simulink model "WK4_FOCIM"  (R2019b)
settings: Solver=VariableStepAuto  StartTime=0.0  StopTime=120.0  MaxStep=1/10000  RelTol=1e-3
values from neighbouring files (symbols this model uses):
  Bm = 15.1e-4    (= 0.00151)    [LAB_FOCIM_sim.m]    (also in LABprep.m; PMAC_machine.m = 7.59908877318e-07; WK1L1_DCmachine.m = Bm_init + Tmax*(i/10)*0.01; WK2_InductionMachine.m = 0.0337986596081)
  CurrentController = tf([133],[1 0])    [LAB_FOCIM_sim.m]    (also in WK4_FOCIM_mScript.m = tf([50],[1 0]))
  Is = 6.3    [LAB_FOCIM_sim.m]    (also in WK4_FOCIM_mScript.m)
  J = 27.6e-3    (= 0.0276)    [LAB_FOCIM_sim.m]    (also in LABprep.m; PMAC_machine.m = 2.55e-08; WK1L1_DCmachine.m = 0.134; WK2_InductionMachine.m = 0.0068)
  La = ((1/Lm)+(1/Lls)+(1/Llrd))^-1    (= 0.0046720399295)    [LAB_FOCIM_sim.m]    (also in LABprep.m = 0.0043; WK2_InductionMachine.m = 0.00475247524752; WK2_InductionMachine_LAB.m = 7.87664870863e-06; WK4_FOCIM_mScript.m = 0.00474852546917)
  Llrd = 11.82e-3    (= 0.01182)    [LAB_FOCIM_sim.m]    (also in WK2_InductionMachine.m = 0.012; WK2_InductionMachine_LAB.m; WK4_FOCIM_mScript.m = 0.012)
  Lls = 7.822*10^-3    (= 0.007822)    [LAB_FOCIM_sim.m]    (also in LABprep.m = 0.007882; PMAC_machine.m = 7.2e-06; WK2_InductionMachine.m = 0.008; WK2_InductionMachine_LAB.m = 7.882e-06)
  Lm = 0.628    [LAB_FOCIM_sim.m]    (also in LABprep.m; PMAC_machine.m = 6.48e-05; WK2_InductionMachine.m = 0.48; WK2_InductionMachine_LAB.m)
  LM_est = 0.9*Lrd_est    (= 0.4428)    [WK4_FOCIM_mScript.m]
  Lrd = Lm + Llrd    (= 0.63982)    [LAB_FOCIM_sim.m]    (also in LABprep.m; WK4_FOCIM_mScript.m = 0.492)
  Lrd_est = Lrd    (= 0.492)    [WK4_FOCIM_mScript.m]
  P = 2    [LAB_FOCIM_sim.m]    (also in PMAC_machine.m; WK2_InductionMachine.m; WK2_InductionMachine_LAB.m; WK4_FOCIM_mScript.m)
  refSpeed = 20    [WK4_FOCIM_mScript.m]
  rrd = 1.868    [LAB_FOCIM_sim.m]    (also in WK2_InductionMachine.m = 1.7; WK2_InductionMachine_LAB.m; WK4_FOCIM_mScript.m = 1.7)
  rs = 1.72    [LAB_FOCIM_sim.m]    (also in WK2_InductionMachine.m = 2; WK2_InductionMachine_LAB.m; WK4_FOCIM_mScript.m = 2)
  SpeedController = tf([0.166],[1 0])    [LAB_FOCIM_sim.m]    (also in WK4_FOCIM_mScript.m)
  w = 0    [LAB_FOCIM_sim.m]    (also in WK2_InductionMachine.m; WK2_InductionMachine_LAB.m; WK4_FOCIM_mScript.m)
libraries: simulink x2
settings Model: Creator=Job  LastModifiedBy=Job
settings DataIOCC: ReturnWorkspaceOutputs=off
settings DebuggingCC: ArithmeticOperatorsInVariantConditions=warning
settings SFSimCC: CustomCodeUndefinedFunction=UseInterfaceOnly

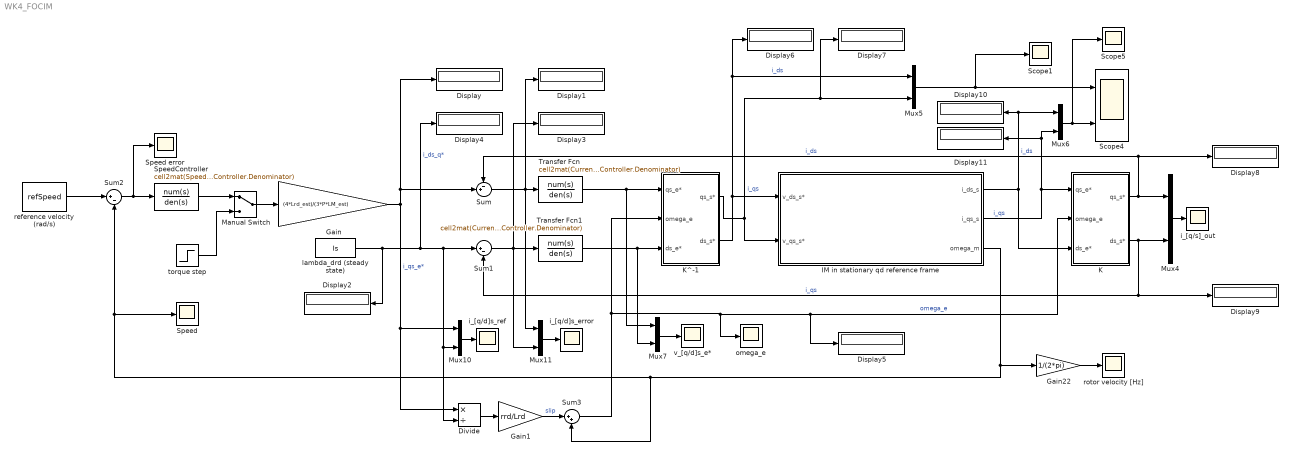
== system WK4_FOCIM ==
  Display{,1..11} (12 alike) : Display
  Divide : Product  Inputs=*/
  Gain : Gain  Gain=(4*Lrd_est)/(3*P*LM_est)
  Gain1 : Gain  Gain=rrd/Lrd
  Gain22 : Gain  Gain=1/(2*pi)
  IM in stationary qd reference frame : Subsystem
  K : Subsystem
  K^-1 : Subsystem
  Manual Switch : ManualSwitch
  Mux{4..7,10..11} (6 alike) : Mux  Inputs=2
  Scope1 : Scope
  Scope4 : Scope  NumInputPorts=2
  Scope5 : Scope
  Speed : Scope
  Speed error : Scope
  SpeedController : TransferFcn  Numerator=cell2mat(SpeedController.Numerator)  Denominator=cell2mat(SpeedController.Denominator)
  Sum : Sum  Inputs=-+|
  Sum1 : Sum  Inputs=|+-
  Sum2 : Sum  Inputs=|+-
  Sum3 : Sum  Inputs=|++
  Transfer Fcn : TransferFcn  Numerator=cell2mat(CurrentController.Numerator)  Denominator=cell2mat(CurrentController.Denominator)
  Transfer Fcn1 : TransferFcn  Numerator=cell2mat(CurrentController.Numerator)  Denominator=cell2mat(CurrentController.Denominator)
  i_[q/d]s_error : Scope
  i_[q/d]s_ref : Scope
  i_[q/s]_out : Scope
  lambda_drd (steady state) : Constant  Value=Is
  omega_e : Scope
  reference velocity (rad/s) : Constant  Value=refSpeed
  rotor velocity [Hz] : Scope
  torque step : Step  Time=20  SampleTime=0
  v_[q/d]s_e* : Scope
  wires:
  Mux4/1 -> i_[q/s]_out/1
  K/1(qs_s*) -> Display8/1, Sum/1, Mux4/1  "i_ds"
  K/2(ds_s*) -> Display9/1, Sum1/2, Mux4/2  "i_qs"
  Gain/1 -> Sum/2, Display/1, Mux10/1, Divide/1  "i_qs_e*"
  lambda_drd (steady state)/1 -> Display2/1, Divide/2, Mux10/2, Sum1/1, Display4/1  "i_ds_q*"
  Sum/1 -> Mux11/1, Display1/1, Transfer Fcn/1
  Sum1/1 -> Mux11/2, Display3/1, Transfer Fcn1/1
  Transfer Fcn1/1 -> Mux7/2, K^-1/3(ds_e*)
  IM in stationary qd reference frame/1(i_ds_s) -> K/3(ds_e*), Display10/1, Mux6/1  "i_ds"
  IM in stationary qd reference frame/2(i_qs_s) -> K/1(qs_e*), Display11/1, Mux6/2  "i_qs"
  Manual Switch/1 -> Gain/1
  IM in stationary qd reference frame/3(omega_m) -> Sum3/2, Speed/1, Sum2/2, Gain22/1
  K^-1/2(ds_s*) -> Display6/1, Mux5/1, IM in stationary qd reference frame/1(v_ds_s*)  "i_ds"
  Mux5/1 -> Scope1/1, Scope4/1
  K^-1/1(qs_s*) -> IM in stationary qd reference frame/2(v_qs_s*), Display7/1, Mux5/2  "i_qs"
  Mux6/1 -> Scope5/1, Scope4/2
  Mux7/1 -> v_[q/d]s_e*/1
  Transfer Fcn/1 -> K^-1/1(qs_e*), Mux7/1
  torque step/1 -> Manual Switch/2
  Sum2/1 -> Speed error/1, SpeedController/1
  SpeedController/1 -> Manual Switch/1
  reference velocity (rad/s)/1 -> Sum2/1
  Mux10/1 -> i_[q/d]s_ref/1
  Mux11/1 -> i_[q/d]s_error/1
  Sum3/1 -> K^-1/2(omega_e), omega_e/1, K/2(omega_e), Display5/1  "omega_e"
  Divide/1 -> Gain1/1
  Gain1/1 -> Sum3/1  "slip"
  Gain22/1 -> rotor velocity [Hz]/1

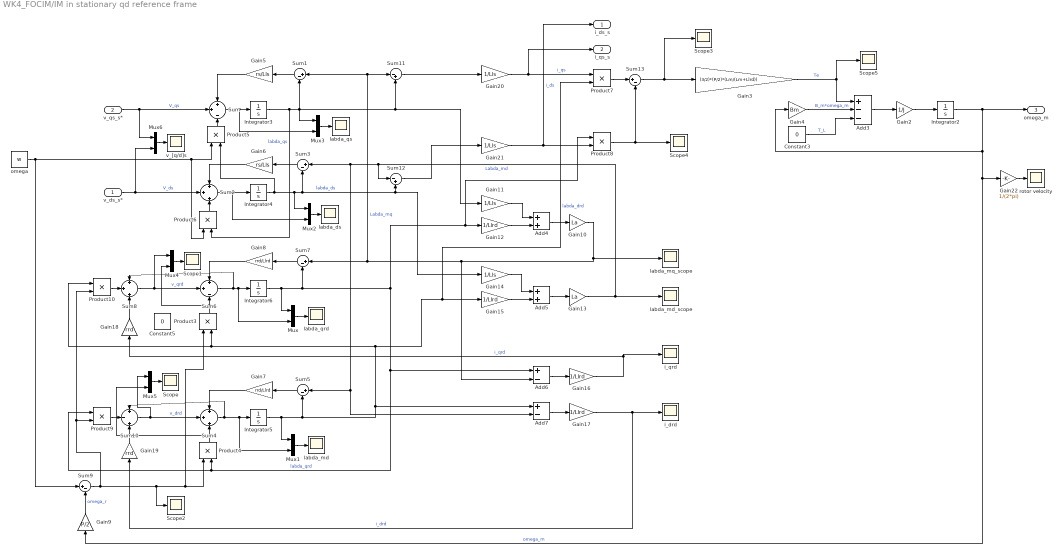
== system WK4_FOCIM/IM in stationary qd reference frame ==
  v_ds_s* : Inport
  v_qs_s* : Inport  Port=2
  Add3 : Sum  Inputs=+--
  Add4 : Sum
  Add5 : Sum
  Add6 : Sum  Inputs=+-
  Add7 : Sum  Inputs=+-
  Constant3 : Constant  Value=0
  Constant5 : Constant  Value=0
  Gain10 : Gain  Gain=La
  Gain{11,14,20..21} (4 alike) : Gain  Gain=1/Lls
  Gain{12,15..17} (4 alike) : Gain  Gain=1/Llrd
  Gain13 : Gain  Gain=La
  Gain18 : Gain  Gain=rrd
  Gain19 : Gain  Gain=rrd
  Gain2 : Gain  Gain=1/J
  Gain22 : Gain  Gain=1/(2*pi)
  Gain3 : Gain  Gain=(3/2)*(P/2)*(Lm/(Lm+Llrd))
  Gain4 : Gain  Gain=Bm
  Gain5 : Gain  Gain=rs/Lls
  Gain6 : Gain  Gain=rs/Lls
  Gain7 : Gain  Gain=rrd/Llrd
  Gain8 : Gain  Gain=rrd/Llrd
  Gain9 : Gain  Gain=P/2
  Integrator{2..6} (5 alike) : Integrator
  Mux{,1..6} (7 alike) : Mux  Inputs=2
  Product{3..10} (8 alike) : Product
  Scope{,1..5} (6 alike) : Scope
  Sum : Sum  Inputs=+|+|-
  Sum{1,3,5,7,9,13} (6 alike) : Sum  Inputs=|+-
  Sum10 : Sum  Inputs=+|-|+
  Sum11 : Sum  Inputs=|-+
  Sum12 : Sum  Inputs=|-+
  Sum2 : Sum  Inputs=+|+|+
  Sum4 : Sum  Inputs=+|+|+
  Sum6 : Sum  Inputs=+|+|-
  Sum8 : Sum  Inputs=+|+|+
  i_drd : Scope
  i_qrd : Scope
  labda_ds : Scope
  labda_md : Scope
  labda_md_scope : Scope
  labda_mq_scope : Scope
  labda_qrd : Scope
  labda_qs : Scope
  omega : Constant  Value=w
  rotor velocity : Scope
  v_[q/d]s : Scope
  i_ds_s : Outport  VectorParamsAs1DForOutWhenUnconnected=off
  i_qs_s : Outport  Port=2  VectorParamsAs1DForOutWhenUnconnected=off
  omega_m : Outport  Port=3  VectorParamsAs1DForOutWhenUnconnected=off
  wires:
  Product10/1 -> Sum8/2
  Product9/1 -> Sum10/2
  Sum13/1 -> Scope3/1, Gain3/1
  omega/1 -> Sum9/1, Product6/1, Product5/1
  Gain21/1 -> i_ds_s/1, Product8/2  "i_ds"
  Sum/1 -> Mux3/2, Integrator3/1
  Gain20/1 -> i_qs_s/1, Product7/1  "i_qs"
  Sum12/1 -> Gain21/1
  Product7/1 -> Sum13/1
  Product3/1 -> Mux4/2, Sum6/3
  Gain16/1 -> i_qrd/1, Gain18/1  "i_qrd"
  Integrator6/1 -> Mux/1, Add6/1, Product9/1, Product4/2, Product8/1, Gain12/1, Sum7/2  "labda_qrd"
  Gain19/1 -> Sum10/3
  Product5/1 -> Sum/3
  Gain18/1 -> Sum8/3
  Gain15/1 -> Add5/2
  Gain11/1 -> Add4/1
  Add6/1 -> Gain16/1
  Add7/1 -> Gain17/1
  Integrator3/1 -> Mux3/1, Gain11/1, Sum11/2, Sum1/2, Product6/2  "labda_qs"
  Integrator5/1 -> Mux1/1, Sum5/2, Add7/1, Product7/2, Gain15/1, Product10/1, Product3/2  "labda_drd"
  Sum6/1 -> Mux/2, Integrator6/1, Sum8/1
  Sum7/1 -> Gain8/1
  Sum9/1 -> Product10/2, Product9/2, Scope2/1, Product3/1, Product4/1
  Sum5/1 -> Gain7/1
  Product4/1 -> Mux5/2, Sum4/3
  Add5/1 -> Gain13/1
  Add3/1 -> Gain2/1
  Gain8/1 -> Sum6/1
  Gain13/1 -> labda_md_scope/1, Sum12/1, Add7/2, Sum5/1, Sum3/1  "Labda_md"
  Sum8/1 -> Sum6/2, Mux4/1  "v_qrd"
  Sum11/1 -> Gain20/1
  Constant3/1 -> Add3/3  "T_L"
  Gain12/1 -> Add4/2
  Gain9/1 -> Sum9/2  "omega_r"
  Add4/1 -> Gain10/1
  Gain22/1 -> rotor velocity/1
  Product6/1 -> Sum2/3
  Gain4/1 -> Add3/2  "B_m*omega_m"
  Gain17/1 -> Gain19/1, i_drd/1  "i_drd"
  Gain2/1 -> Integrator2/1
  Sum1/1 -> Gain5/1
  Integrator2/1 -> omega_m/1, Gain22/1, Gain9/1, Gain4/1  "omega_m"
  Product8/1 -> Scope4/1, Sum13/2
  v_ds_s*/1 -> Mux6/2, Sum2/2  "V_ds"
  Sum2/1 -> Mux2/2, Integrator4/1
  Gain6/1 -> Sum2/1
  Gain14/1 -> Add5/1
  Gain7/1 -> Sum4/1
  v_qs_s*/1 -> Mux6/1, Sum/2  "V_qs"
  Gain5/1 -> Sum/1
  Gain10/1 -> labda_mq_scope/1, Add6/2, Sum11/1, Sum1/1, Sum7/1  "Labda_mq"
  Integrator4/1 -> Mux2/1, Sum12/2, Gain14/1, Sum3/2, Product5/2  "labda_ds"
  Sum4/1 -> Sum10/1, Mux1/2, Integrator5/1
  Sum10/1 -> Sum4/2, Mux5/1  "v_drd"
  Sum3/1 -> Gain6/1
  Gain3/1 -> Scope5/1, Add3/1  "Te"
  Mux/1 -> labda_qrd/1
  Mux1/1 -> labda_md/1
  Mux2/1 -> labda_ds/1
  Mux3/1 -> labda_qs/1
  Mux4/1 -> Scope1/1
  Mux5/1 -> Scope/1
  Mux6/1 -> v_[q/d]s/1

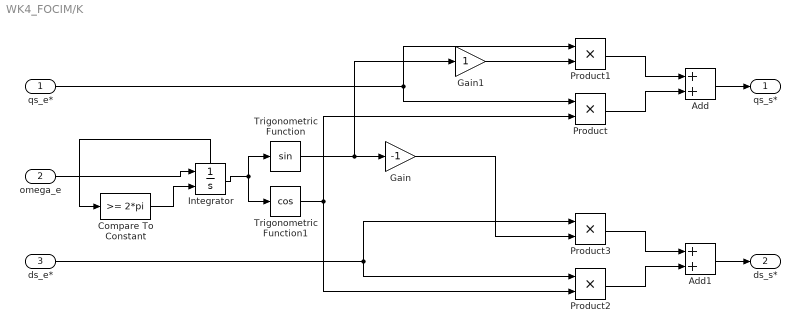
== system WK4_FOCIM/K ==
  qs_e* : Inport
  omega_e : Inport  Port=2
  ds_e* : Inport  Port=3
  Add : Sum
  Add1 : Sum
  Compare To Constant : simulink/Logic and Bit Operations/Compare To Constant  relop=>=  const=2*pi  OutDataTypeStr=boolean
  Gain : Gain  Gain=-1
  Gain1 : Gain
  Integrator : Integrator  ExternalReset=rising  ShowStatePort=on
  Product{,1..3} (4 alike) : Product
  Trigonometric Function : Trigonometry
  Trigonometric Function1 : Trigonometry  Operator=cos
  qs_s* : Outport  VectorParamsAs1DForOutWhenUnconnected=off
  ds_s* : Outport  Port=2  VectorParamsAs1DForOutWhenUnconnected=off
  wires:
  ds_e*/1 -> Product3/1, Product2/1
  Add1/1 -> ds_s*/1
  Product2/1 -> Add1/2
  Product3/1 -> Add1/1
  Trigonometric Function1/1 -> Product/2, Product2/2
  Add/1 -> qs_s*/1
  Product1/1 -> Add/1
  qs_e*/1 -> Product/1, Product1/1
  Trigonometric Function/1 -> Gain1/1, Gain/1
  Integrator/1 -> Trigonometric Function1/1, Trigonometric Function/1
  Product/1 -> Add/2
  omega_e/1 -> Integrator/1
  Compare To Constant/1 -> Integrator/2
  Integrator/State -> Compare To Constant/1
  Gain/1 -> Product3/2
  Gain1/1 -> Product1/2

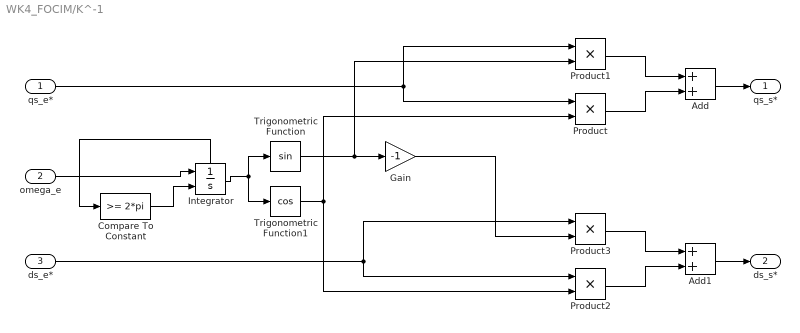
== system WK4_FOCIM/K^-1 ==
  qs_e* : Inport
  omega_e : Inport  Port=2
  ds_e* : Inport  Port=3
  Add : Sum
  Add1 : Sum
  Compare To Constant : simulink/Logic and Bit Operations/Compare To Constant  relop=>=  const=2*pi  OutDataTypeStr=boolean
  Gain : Gain  Gain=-1
  Integrator : Integrator  ExternalReset=rising  ShowStatePort=on
  Product{,1..3} (4 alike) : Product
  Trigonometric Function : Trigonometry
  Trigonometric Function1 : Trigonometry  Operator=cos
  qs_s* : Outport  VectorParamsAs1DForOutWhenUnconnected=off
  ds_s* : Outport  Port=2  VectorParamsAs1DForOutWhenUnconnected=off
  wires:
  ds_e*/1 -> Product3/1, Product2/1
  Add1/1 -> ds_s*/1
  Product2/1 -> Add1/2
  Product3/1 -> Add1/1
  Trigonometric Function1/1 -> Product/2, Product2/2
  Add/1 -> qs_s*/1
  Product1/1 -> Add/1
  qs_e*/1 -> Product/1, Product1/1
  Trigonometric Function/1 -> Product1/2, Gain/1
  Integrator/1 -> Trigonometric Function1/1, Trigonometric Function/1
  Product/1 -> Add/2
  omega_e/1 -> Integrator/1
  Compare To Constant/1 -> Integrator/2
  Integrator/State -> Compare To Constant/1
  Gain/1 -> Product3/2
